simulink model "ProjectLogicGateThreeCoscecutive1's"  (R2018a)
settings: Solver=VariableStepAuto  StartTime=0.0  StopTime=10.0  RelTol=1e-3
settings Model: Creator=Bhaskar  LastModifiedBy=Bhaskar

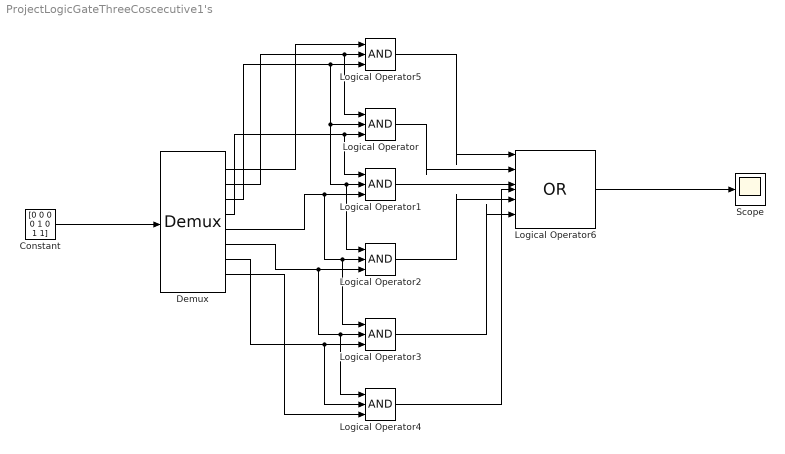
== system ProjectLogicGateThreeCoscecutive1's ==
  Constant : Constant  Value=[0 0 0 0 1 0 1 1]
  Demux : Demux  Outputs=8
  Logical Operator{,1..5} (6 alike) : Logic  Inputs=3  IconShape=distinctive  AllPortsSameDT=off  OutDataTypeStr=boolean
  Logical Operator6 : Logic  Operator=OR  Inputs=6  IconShape=distinctive  AllPortsSameDT=off  OutDataTypeStr=boolean
  Scope : Scope
  wires:
  Constant/1 -> Demux/1
  Demux/1 -> Logical Operator5/1
  Demux/2 -> Logical Operator/1, Logical Operator5/2
  Demux/3 -> Logical Operator2/1, Logical Operator1/2, Logical Operator/2, Logical Operator5/3
  Demux/4 -> Logical Operator1/1, Logical Operator/3
  Demux/5 -> Logical Operator3/1, Logical Operator2/2, Logical Operator1/3
  Demux/6 -> Logical Operator4/1, Logical Operator3/2, Logical Operator2/3
  Demux/7 -> Logical Operator4/2, Logical Operator3/3
  Demux/8 -> Logical Operator4/3
  Logical Operator5/1 -> Logical Operator6/1
  Logical Operator/1 -> Logical Operator6/2
  Logical Operator1/1 -> Logical Operator6/3
  Logical Operator2/1 -> Logical Operator6/4
  Logical Operator3/1 -> Logical Operator6/5
  Logical Operator4/1 -> Logical Operator6/6
  Logical Operator6/1 -> Scope/1
